simulink model "BACKADAPTATIVE"  (R2024a)
settings: Solver=VariableStepAuto  StartTime=0.0  StopTime=50  RelTol=1e-3
settings Model: Creator=VICTUS  LastModifiedBy=VICTUS

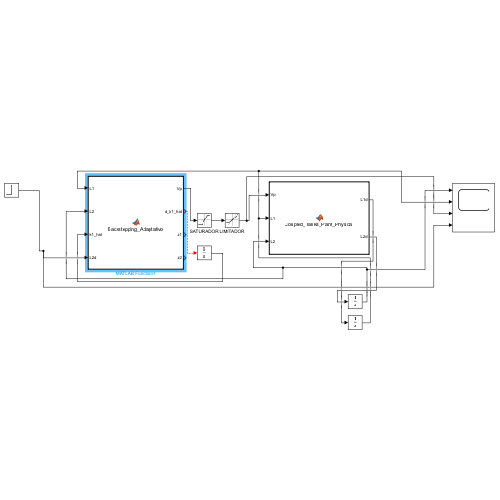
[thumbnail: Simulink's stored preview of the top-level diagram]
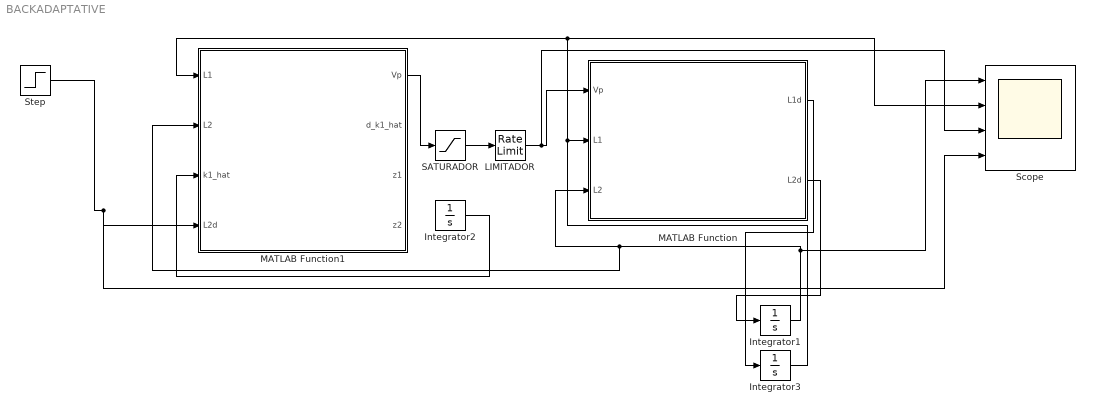
== system BACKADAPTATIVE ==
  Integrator1 : Integrator
  Integrator2 : Integrator
  Integrator3 : Integrator
  LIMITADOR : RateLimiter  RisingSlewLimit=50  FallingSlewLimit=-50  SampleTimeMode=inherited
  MATLAB Function : MATLAB Function  TreatAsAtomicUnit=on
  MATLAB Function1 : MATLAB Function  TreatAsAtomicUnit=on
  SATURADOR : Saturate  UpperLimit=22  LowerLimit=0
  Scope : Scope  NumInputPorts=4
  Step : Step  Time=0  After=10  SampleTime=0.001
  wires:
  LIMITADOR/1 -> Scope/3, MATLAB Function/1(Vp)
  SATURADOR/1 -> LIMITADOR/1
  MATLAB Function1/1(Vp) -> SATURADOR/1
  Step/1 -> Scope/4, MATLAB Function1/4(L2d)
  MATLAB Function/1(L1d) -> Integrator3/1
  Integrator3/1 -> Scope/2, MATLAB Function1/1(L1), MATLAB Function/2(L1)
  MATLAB Function/2(L2d) -> Integrator1/1
  ? -> Integrator2/1
  Integrator2/1 -> MATLAB Function1/3(k1_hat)
  Integrator1/1 -> Scope/1, MATLAB Function1/2(L2), MATLAB Function/3(L2)

== matlab function BACKADAPTATIVE/MATLAB Function1 ==
  data: L1 input; Vp output; L2 input; k1_hat input; L2d input; d_k1_hat output; z1 output; z2 output
function [Vp, d_k1_hat, z1, z2] = Backstepping_Adaptativo(L1, L2, k1_hat, L2d)
% Controlador Backstepping Adaptativo (Estima solo k1)

    
% Parámetros Físicos 
%% ===== PARÁMETROS FÍSICOS DEL SISTEMA =====
dt1 = 4.445;   % diámetro tanque 1 [cm]
dt2 = 4.445;   % diámetro tanque 2 [cm]
d01 = 0.635;   % diámetro orificio tanque 1 [cm]
d02 = 0.47625; % diámetro orificio tanque 2 [cm]
At1 = pi*(dt1^2)/4;   % área transversal tanque 1 [cm²]
At2 = pi*(dt2^2)/4;   % área transversal tanque 2 [cm²]
Ao1 = pi*(d01^2)/4;   % área orificio tanque 1 [cm²]
Ao2 = pi*(d02^2)/4;   % área orificio tanque 2 [cm²]
g  = 981;              % gravedad [cm/s²]

% Parámetros del Modelo (k2, k3, k4 se asumen conocidos)
k2 = (Ao1 * sqrt(2*g)) / At1; % (aprox 0.9031)
k3 = (Ao1 * sqrt(2*g)) / At2; % (aprox 0.9031)
k4 = (Ao2 * sqrt(2*g)) / At2; % (aprox 0.9031)

% Ganancias del Controlador (Puedes necesitar AJUSTARLAS)
c1 = 0.5;       % Velocidad de z1 (L2)
c2 = 1.5;       % Velocidad de z2 (L1)
gamma1 = 0.01;   % Velocidad de adaptación de k1_hat (Aumentada de 0.01)

% Límites
Vp_max = 22.0;  %
Vp_min = 0.0;   %
k1_hat_min = 0.01; % Proyección para evitar división por cero

% --- 1.5. INICIALIZACIÓN DE SALIDAS ---
Vp = 0.0;
d_k1_hat = 0.0;
z1 = 0.0;
z2 = 0.0;

% --- 2. Protecciones Numéricas ---
epsilon = 1e-6; 
L1_safe = max(L1, epsilon);
L2_safe = max(L2, epsilon);
sqrt_L1_safe = sqrt(L1_safe);
sqrt_L2_safe = sqrt(L2_safe);
k1_hat_safe = max(k1_hat, k1_hat_min);

% --- 3. PASO 1: Diseño No Adaptativo para L2 ---
z1 = L2 - L2d;
alpha1 = (1/k3) * (k4 * sqrt_L2_safe - c1 * z1);
z2 = sqrt_L1_safe - alpha1;

% --- 4. PASO 2: Diseño Adaptativo para L1 ---

% Cálculo de d_alpha1
d_alpha1_d_L2 = (1/k3) * (k4 / (2*sqrt_L2_safe) - c1);
dL2 = k3 * sqrt_L1_safe - k4 * sqrt_L2_safe; 
d_alpha1 = d_alpha1_d_L2 * dL2;


% 4.a. Definir el término 'Phi' (el contenido del paréntesis)
Phi = -c2*z2 - k3*z1 + k2/2 + d_alpha1;

% 4.b. Ley de Control Vp (basada en Phi)
Vp = (2*sqrt_L1_safe / k1_hat_safe) * Phi;

% 4.c. Ley de Actualización (basada en Phi, numéricamente estable)
% Esta es la corrección principal: no hay división por sqrt(L1)
d_k1_hat = (gamma1 * z2 * Phi) / k1_hat_safe;

== matlab function BACKADAPTATIVE/MATLAB Function ==
  data: Vp input; L1d output; L2d output; L1 input; L2 input
function [L1d, L2d] = Coupled_Tanks_Plant_Physical(Vp,L1, L2)
% Modelo no lineal simplificado de tanques acoplados Quanser

dt1 = 4.445; dt2 = 4.445;
d01 = 0.635; d02 = 0.47625;
At1 = pi*(dt1^2)/4;  At2 = pi*(dt2^2)/4;
Ao1 = pi*(d01^2)/4;  Ao2 = pi*(d02^2)/4;
Kp = 3.3;  g = 981;


Fin = Kp * Vp;
Fout1 = Ao1 * sqrt(2*g*L1);
Fout2 = Ao2 * sqrt(2*g*L2);
F12 = Fout1;

L1d = (Fin - Fout1) / At1;
L2d = (F12 - Fout2) / At2;
end
